simulink subsystem "rss_ParkTrasfSens"  (R2023a)
settings: Solver=VariableStepAuto  StartTime=0.0  StopTime=5  RelTol=1e-3
undefined symbols (not defined in the file): Cdbl_iPhCurrMaxVal, Cdbl_nElecAgSpdMaxVal, Cdbl_nElecAgSpdPeakVal, Cdbl_uPhVltgMaxVal, ENM_MOTO_STATUS, Gs16_tCtlVltgDelTi_C
libraries: lib_conversion x2, lib_park_transform x2, simulink x1
settings Model: DefaultTestHarness=rss_ParkTransform_SensorBased_thu  Creator=RAN2OFO  LastModifiedBy=xiaoqiang.yuan
settings OptimizationCC: ReuseModelBlockBuffer=off

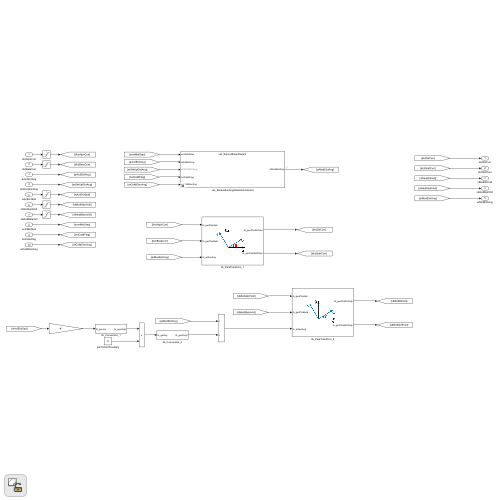
[thumbnail: Simulink's stored preview of the top-level diagram]
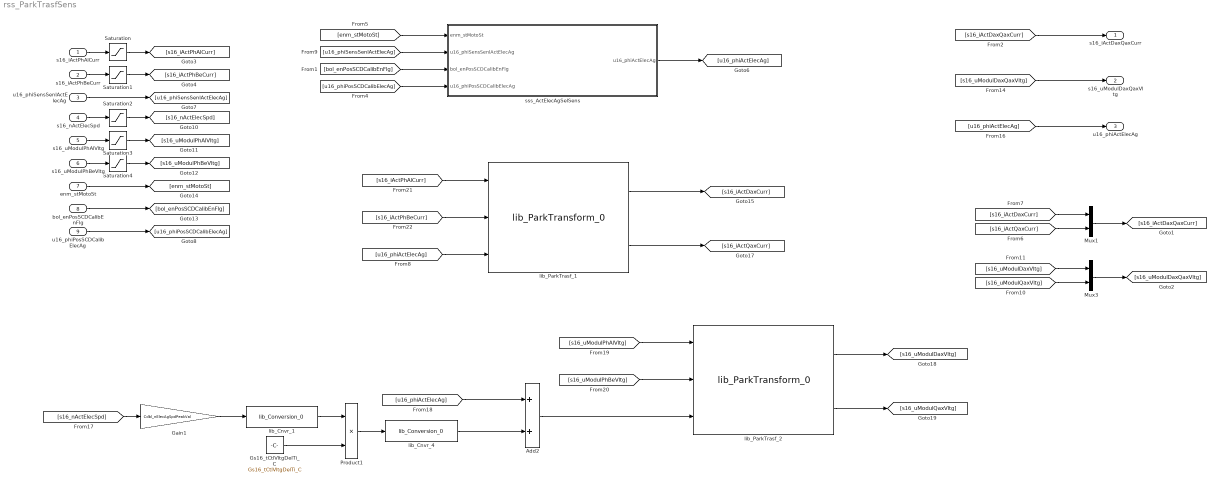
== system rss_ParkTrasfSens ==
  s16_iActPhAlCurr : Inport  OutDataTypeStr=dt_Standardize_s16p15b0
  s16_iActPhBeCurr : Inport  Port=2  OutDataTypeStr=dt_Standardize_s16p15b0
  u16_phiSensSenlActElecAg : Inport  Port=3  OutDataTypeStr=dt_RadAng_u16r15b0
  s16_nActElecSpd : Inport  Port=4  OutDataTypeStr=dt_Standardize_s16p15b0
  s16_uModulPhAlVltg : Inport  Port=5  OutDataTypeStr=dt_Standardize_s16p15b0
  s16_uModulPhBeVltg : Inport  Port=6  OutDataTypeStr=dt_Standardize_s16p15b0
  enm_stMotoSt : Inport  Port=7  OutDataTypeStr=Enum: ENM_MOTO_STATUS
  bol_enPosSCDCalibEnFlg : Inport  Port=8  OutDataTypeStr=boolean
  u16_phiPosSCDCalibElecAg : Inport  Port=9  OutDataTypeStr=dt_RadAng_u16r15b0
  Add2 : Sum  InitFcn=|  OutDataTypeStr=Inherit: Same as first input
      | Simulink.suppressDiagnostic(gcb,...
      | 'SimulinkFixedPoint:util:Overflowoccurred');
  Gain1 : Gain  Gain=Cdbl_nElecAgSpdPeakVal  OutDataTypeStr=Inherit: Inherit via back propagation
  Gs16_tCtlVltgDelTi_C : Constant  Value=Gs16_tCtlVltgDelTi_C
  Mux1 : Mux  Inputs=2
  Mux3 : Mux  Inputs=2
  Product1 : Product  OutDataTypeStr=Inherit: Inherit via back propagation
  Saturation : Saturate  UpperLimit=Cdbl_iPhCurrMaxVal  LowerLimit=-Cdbl_iPhCurrMaxVal
  Saturation1 : Saturate  UpperLimit=Cdbl_iPhCurrMaxVal  LowerLimit=-Cdbl_iPhCurrMaxVal
  Saturation2 : Saturate  UpperLimit=Cdbl_nElecAgSpdMaxVal  LowerLimit=-Cdbl_nElecAgSpdMaxVal
  Saturation3 : Saturate  UpperLimit=Cdbl_uPhVltgMaxVal  LowerLimit=-Cdbl_uPhVltgMaxVal
  Saturation4 : Saturate  UpperLimit=Cdbl_uPhVltgMaxVal  LowerLimit=-Cdbl_uPhVltgMaxVal
  lib_Cnvr_1 : lib_conversion/lib_Conversion_0  lb_parDataType=fixdt(1,16)  lb_parOutpMaxVal=Cdbl_nElecAgSpdPeakVal  lb_parOutpMinVal=[]  lb_parSatFlag=off
  lib_Cnvr_4 : lib_conversion/lib_Conversion_0  lb_parDataType=fixdt(1,16,pi*2^-15,0)  lb_parOutpMaxVal=[]  lb_parOutpMinVal=[]  lb_parSatFlag=off
  lib_ParkTrasf_1 : lib_park_transform/lib_ParkTransform_0  VariantControl=ClarkTransf_MIL_flo  lb_parSelRotFrmeAxis=d-axis
  lib_ParkTrasf_2 : lib_park_transform/lib_ParkTransform_0  VariantControl=ClarkTransf_MIL_flo  lb_parSelRotFrmeAxis=d-axis
  sss_ActElecAgSelSens : Subsystem  VariantControl=cstSensCtrlLbl
  s16_iActDaxQaxCurr : Outport  OutDataTypeStr=dt_Standardize_s16p15b0
  s16_uModulDaxQaxVltg : Outport  Port=2  OutDataTypeStr=dt_Standardize_s16p15b0
  u16_phiActElecAg : Outport  Port=3  OutDataTypeStr=dt_RadAng_u16r15b0
  wires:
  [s16_uModulDaxQaxVltg] -> s16_uModulDaxQaxVltg/1
  s16_uModulPhBeVltg/1 -> Saturation4/1
  s16_uModulPhAlVltg/1 -> Saturation3/1
  Saturation3/1 -> [s16_uModulPhAlVltg]
  Saturation4/1 -> [s16_uModulPhBeVltg]
  Saturation2/1 -> [s16_nActElecSpd]
  [s16_iActDaxQaxCurr] -> s16_iActDaxQaxCurr/1
  Saturation/1 -> [s16_iActPhAlCurr]
  s16_iActPhAlCurr/1 -> Saturation/1
  u16_phiSensSenlActElecAg/1 -> [u16_phiSensSenlActElecAg]
  s16_iActPhBeCurr/1 -> Saturation1/1
  s16_nActElecSpd/1 -> Saturation2/1
  Saturation1/1 -> [s16_iActPhBeCurr]
  [u16_phiPosSCDCalibElecAg] -> sss_ActElecAgSelSens/4(u16_phiPosSCDCalibElecAg)
  [enm_stMotoSt] -> sss_ActElecAgSelSens/1(enm_stMotoSt)
  [u16_phiSensSenlActElecAg] -> sss_ActElecAgSelSens/2(u16_phiSensSenlActElecAg)
  [bol_enPosSCDCalibEnFlg] -> sss_ActElecAgSelSens/3(bol_enPosSCDCalibEnFlg)
  u16_phiPosSCDCalibElecAg/1 -> [u16_phiPosSCDCalibElecAg]
  bol_enPosSCDCalibEnFlg/1 -> [bol_enPosSCDCalibEnFlg]
  enm_stMotoSt/1 -> [enm_stMotoSt]
  sss_ActElecAgSelSens/1(u16_phiActElecAg) -> [u16_phiActElecAg]
  [u16_phiActElecAg] -> u16_phiActElecAg/1
  [s16_uModulPhAlVltg] -> lib_ParkTrasf_2/1
  [u16_phiActElecAg] -> lib_ParkTrasf_1/3
  Gain1/1 -> lib_Cnvr_1/1
  lib_Cnvr_1/1 -> Product1/1
  Gs16_tCtlVltgDelTi_C/1 -> Product1/2
  Add2/1 -> lib_ParkTrasf_2/3
  lib_ParkTrasf_1/2 -> [s16_iActQaxCurr]
  [s16_nActElecSpd] -> Gain1/1
  lib_ParkTrasf_2/1 -> [s16_uModulDaxVltg]
  [s16_uModulPhBeVltg] -> lib_ParkTrasf_2/2
  lib_ParkTrasf_2/2 -> [s16_uModulQaxVltg]
  [u16_phiActElecAg] -> Add2/1
  lib_ParkTrasf_1/1 -> [s16_iActDaxCurr]
  [s16_iActPhBeCurr] -> lib_ParkTrasf_1/2
  Product1/1 -> lib_Cnvr_4/1
  lib_Cnvr_4/1 -> Add2/2
  [s16_iActPhAlCurr] -> lib_ParkTrasf_1/1
  [s16_uModulQaxVltg] -> Mux3/2
  Mux1/1 -> [s16_iActDaxQaxCurr]
  [s16_iActDaxCurr] -> Mux1/1
  [s16_iActQaxCurr] -> Mux1/2
  Mux3/1 -> [s16_uModulDaxQaxVltg]
  [s16_uModulDaxVltg] -> Mux3/1

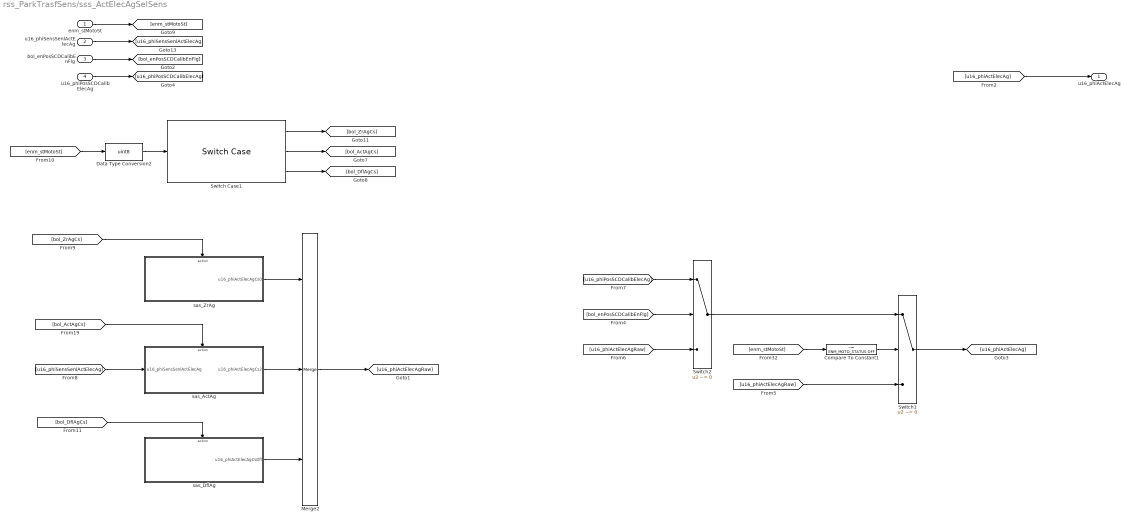
== system rss_ParkTrasfSens/sss_ActElecAgSelSens ==
  enm_stMotoSt : Inport
  u16_phiSensSenlActElecAg : Inport  Port=2
  bol_enPosSCDCalibEnFlg : Inport  Port=3
  u16_phiPosSCDCalibElecAg : Inport  Port=4
  Compare To Constant1 : simulink/Logic and Bit Operations/Compare To Constant  relop=~=  const=ENM_MOTO_STATUS.OFF  OutDataTypeStr=boolean
  Data Type Conversion2 : DataTypeConversion  OutDataTypeStr=uint8  SaturateOnIntegerOverflow=off  RndMeth=Floor
  Merge2 : Merge  Inputs=3
  Switch Case1 : SwitchCase  CaseConditions={0,2}
  Switch1 : Switch  Criteria=u2 ~= 0  SaturateOnIntegerOverflow=off  InputSameDT=off
  Switch2 : Switch  Criteria=u2 ~= 0  SaturateOnIntegerOverflow=off  InputSameDT=off
  sas_ActAg : Subsystem  TreatAsAtomicUnit=on
  sas_DflAg : Subsystem  TreatAsAtomicUnit=on
  sas_ZrAg : Subsystem  TreatAsAtomicUnit=on
  u16_phiActElecAg : Outport
  wires:
  sas_ActAg/1(u16_phiActElecAgCs2) -> Merge2/2
  sas_DflAg/1(u16_phiActElecAgCsDfl) -> Merge2/3
  Switch Case1/1 -> [bol_ZrAgCs]
  Merge2/1 -> [u16_phiActElecAgRaw]
  Switch Case1/2 -> [bol_ActAgCs]
  [bol_ZrAgCs] -> sas_ZrAg/Action
  [enm_stMotoSt] -> Data Type Conversion2/1
  sas_ZrAg/1(u16_phiActElecAgCs0) -> Merge2/1
  Switch Case1/3 -> [bol_DflAgCs]
  [u16_phiSensSenlActElecAg] -> sas_ActAg/1(u16_phiSensSenlActElecAg)
  [bol_ActAgCs] -> sas_ActAg/Action
  Data Type Conversion2/1 -> Switch Case1/1
  [bol_DflAgCs] -> sas_DflAg/Action
  u16_phiPosSCDCalibElecAg/1 -> [u16_phiPosSCDCalibElecAg]
  [u16_phiPosSCDCalibElecAg] -> Switch2/1
  [u16_phiActElecAgRaw] -> Switch2/3
  Switch2/1 -> Switch1/1
  [u16_phiActElecAgRaw] -> Switch1/3
  [bol_enPosSCDCalibEnFlg] -> Switch2/2
  Switch1/1 -> [u16_phiActElecAg]
  Compare To Constant1/1 -> Switch1/2
  [enm_stMotoSt] -> Compare To Constant1/1
  bol_enPosSCDCalibEnFlg/1 -> [bol_enPosSCDCalibEnFlg]
  enm_stMotoSt/1 -> [enm_stMotoSt]
  u16_phiSensSenlActElecAg/1 -> [u16_phiSensSenlActElecAg]
  [u16_phiActElecAg] -> u16_phiActElecAg/1

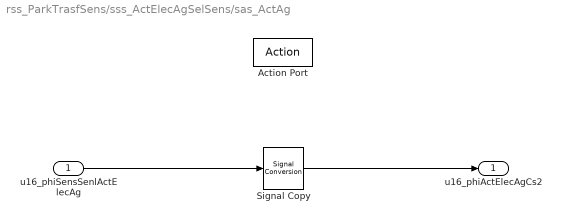
== system rss_ParkTrasfSens/sss_ActElecAgSelSens/sas_ActAg ==
  u16_phiSensSenlActElecAg : Inport
  Action Port : ActionPort
  Signal Copy : SignalConversion  OverrideOpt=off
  u16_phiActElecAgCs2 : Outport
  wires:
  Signal Copy/1 -> u16_phiActElecAgCs2/1
  u16_phiSensSenlActElecAg/1 -> Signal Copy/1

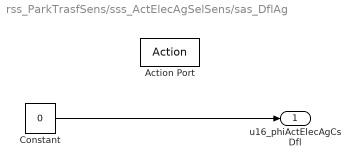
== system rss_ParkTrasfSens/sss_ActElecAgSelSens/sas_DflAg ==
  Action Port : ActionPort
  Constant : Constant  Value=0  OutDataTypeStr=dt_RadAng_u16r15b0
  u16_phiActElecAgCsDfl : Outport
  wires:
  Constant/1 -> u16_phiActElecAgCsDfl/1

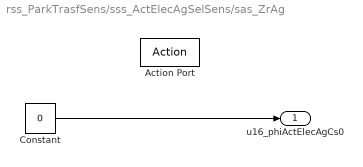
== system rss_ParkTrasfSens/sss_ActElecAgSelSens/sas_ZrAg ==
  Action Port : ActionPort
  Constant : Constant  Value=0  OutDataTypeStr=dt_RadAng_u16r15b0
  u16_phiActElecAgCs0 : Outport
  wires:
  Constant/1 -> u16_phiActElecAgCs0/1
